simulink model "expo_proj"  (R2023b)
settings: Solver=FixedStepAuto  StartTime=0.0  StopTime=999  RelTol=1e-3  EnableMultiTasking=on
libraries: stm32f4xxblockslib x3, stm32blockslib x1
settings Model: SimulationMode=external  ExtModeTrigDuration=10  Creator=Aidan  LastModifiedBy=Aidan
settings OptimizationCC: EnhancedBackFolding=on  PassReuseOutputArgsAs=Individual arguments  ZeroExternalMemoryAtStartup=off  ZeroInternalMemoryAtStartup=off  MaxStackSize=64  OptimizeBlockOrder=speed  DifferentSizesBufferReuse=on  OptimizationCustomize=off  EfficientTunableParamExpr=on
settings DebuggingCC: ParameterTunabilityLossMsg=error
settings HardwareCC: ProdBitPerPointer=32  ProdBitPerSizeT=32  ProdBitPerPtrDiffT=32  ProdLargestAtomicInteger=Long  ProdLargestAtomicFloat=Double  ProdWordSize=32  ProdLongLongMode=on  ProdHWDeviceType=ARM Compatible->ARM Cortex
settings SFSimCC: MATLABDynamicMemAlloc=off
settings RTWCC: Description=Embedded Coder  SystemTargetFile=ert.tlc  HardwareBoard=STM32F7xx Based (Single precision FPU)  TemplateMakefile=ert_default_tmf  Toolchain=GNU Tools for ARM Embedded Processors
settings CodeAppCC: ForceParamTrailComments=on  IgnoreCustomStorageClasses=off  OperatorAnnotations=on  SimulinkDataObjDesc=on  SFDataObjDesc=on  InsertBlockDesc=on
settings ERTTargetCC: CodeReplacementLibrary=ARM Cortex-M  ExtModeTransport=3  ExtModeStaticAlloc=on  ExtModeStaticAllocSize=2048  ExtModeMexFile=ext_xcp  ExtModeIntrfLevel=Level2 - Open

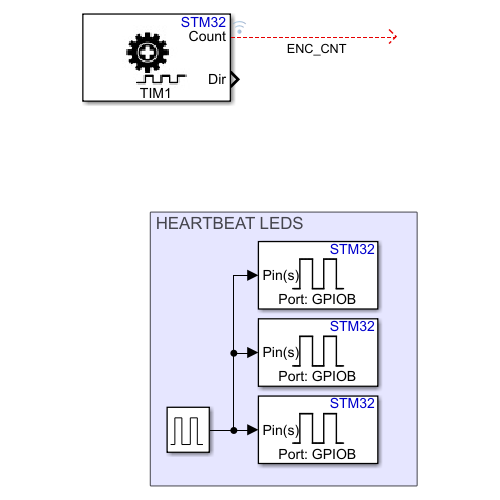
[thumbnail: Simulink's stored preview of the top-level diagram]
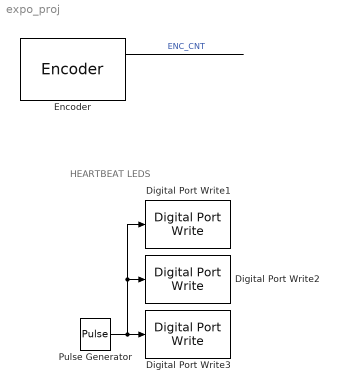
== system expo_proj ==
  note: HEARTBEAT LEDS
  Digital Port Write1 : stm32f4xxblockslib/Digital Port Write  PortName=GPIOB  PinNumber=[0]  ReadOperation=off  IOAsArray=on  EnableSimPort=off
      settings: LibrarySourceBlock=stm32f7xxblockslib/Digital Port Write
  Digital Port Write2 : stm32f4xxblockslib/Digital Port Write  PortName=GPIOB  PinNumber=[14]  ReadOperation=off  IOAsArray=on  EnableSimPort=off
      settings: LibrarySourceBlock=stm32f7xxblockslib/Digital Port Write
  Digital Port Write3 : stm32f4xxblockslib/Digital Port Write  PortName=GPIOB  PinNumber=[7]  ReadOperation=off  IOAsArray=on  EnableSimPort=off
      settings: LibrarySourceBlock=stm32f7xxblockslib/Digital Port Write
  Encoder : stm32blockslib/Encoder  TimerModule=TIM1  EnableResetInput=off  OutputDirection=on  SampleTime=-1
      settings: LibrarySourceBlock=stm32f7xxblockslib/Encoder
  Pulse Generator : DiscretePulseGenerator  PulseType=Time based  Period=1  PulseWidth=50  SampleTime=0.1
  wires:
  Pulse Generator/1 -> Digital Port Write3/1, Digital Port Write2/1, Digital Port Write1/1
  Encoder/1 -> ?  "ENC_CNT"
